simulink model "Lab6_dysk_PID"  (R2017a)
settings: Solver=VariableStepAuto  StartTime=0.0  StopTime=10.0  FixedStep=0.1  MaxStep=0.1  RelTol=1e-3
values from neighbouring files (symbols this model uses):
  h = bodeplot(K)    [Lab1.m]    (also in Lab5.m = nyquistplot(K0); Lab6.m = h1)
libraries: cstblocks x2
settings Model: Creator=ishiguro  LastModifiedBy=ishiguro
settings DataIOCC: TimeSaveName=tout_PID

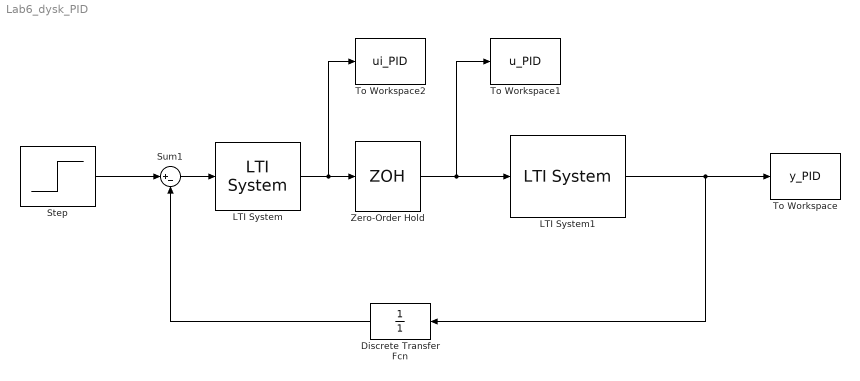
== system Lab6_dysk_PID ==
  Discrete Transfer Fcn : DiscreteTransferFcn  Denominator=[1]  SampleTime=h
  LTI System : cstblocks/LTI System  sys=Hr  IC=[]
  LTI System1 : cstblocks/LTI System  sys=K  IC=[]
  Step : Step  Time=0  SampleTime=0
  Sum1 : Sum  Inputs=|+-
  To Workspace : ToWorkspace  VariableName=y_PID  SampleTime=-1
  To Workspace1 : ToWorkspace  VariableName=u_PID  SampleTime=-1
  To Workspace2 : ToWorkspace  VariableName=ui_PID  SaveFormat=Structure With Time  SampleTime=-1
  Zero-Order Hold : ZeroOrderHold  SampleTime=h
  wires:
  LTI System/1 -> To Workspace2/1, Zero-Order Hold/1
  Discrete Transfer Fcn/1 -> Sum1/2
  Sum1/1 -> LTI System/1
  LTI System1/1 -> Discrete Transfer Fcn/1, To Workspace/1
  Step/1 -> Sum1/1
  Zero-Order Hold/1 -> To Workspace1/1, LTI System1/1
